simulink library "SMC"  (R2019a)
settings: Solver=VariableStepAuto  StartTime=0.0  StopTime=10.0  RelTol=1e-3
values from neighbouring files (symbols this model uses):
  A = BWB.lat.A    [Example_init.m]    (also in SMC1.m = BWB.A; SMCCanForm.m = Tr*A*Tr')
  B = BWB.lat.B    [Example_init.m]    (also in SMC1.m = BWB.B; SMCCanForm.m = Tr*B)
  CA = pinv(B2)    [SMCCanForm.m]
  Cc = [1 0 0 0 ... (first row only)    [Example_init.m]    (also in outfor.m = C*inv(Tc))
  F = -eye(2)    [Example_init.m]    (also in sqobs.m = (P2*C2*B2)')
  Lam = S*Bf    [comrobs.m]    (also in contl.m = S*B; contlCA.m = S*B; contliaCA.m = S*BT; contliaCA2.m = S*BT)
  P = lyap(Phi',eye(mm))    [comrobs.m]    (also in contl.m; contlCA.m; contliaCA.m; contliaCA2.m)
  Q = eye(4)    [Example_init.m]
  Qi = eye(2)    [Example_init.m]
settings Model: Creator=lev201  LastModifiedBy=Witali
settings DataIOCC: ReturnWorkspaceOutputs=off
settings DebuggingCC: ArithmeticOperatorsInVariantConditions=warning
settings SFSimCC: SimUseLocalCustomCode=off
settings RTWCC: RTWUseLocalCustomCode=off

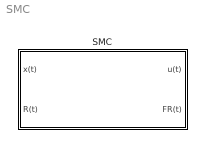
== system SMC ==
  SMC : Subsystem  mask{I=on, shs=off, adpt=off, showadpt=off, A=A, B=B, Cc=Cc, Q=Q, rho=1, C0=1, PC=1, K0=1, PK=1, delta=0.01, eps=0, Qi=Qi, Fil=on, Filter=F, FRt=on}
      mask prompts: I "Integral Action"; shs "Show s(t)"; adpt "Adaptive"; showadpt "Show Adaptive Parameters"; A "System Matrix:"; B "Effectiveness Matrix:"; Cc "Output Matrix:"; Q "State Weighting Matrix:"; C0 "Initial guess of C:"; PC "Learning rate of C estimator:"; K0 "Initial guess of K:"; PK "Learning rate of K estimator:"; delta "Sigmoidal Approximation:"; eps "Boundary Layer Thickness:"; Qi "Integral Action Weighting Matrix:"; Fil "Pre-Filter Reference Signal"; FRt "Show Filtered R(t)"
      mask init:
      | Shs=get_param(gcb, 'shs');
      | int=get_param(gcb, 'I');
      | Fil=get_param(gcb, 'fil');
      | FRT=get_param(gcb, 'FRt');
      | SAD=get_param(gcb, 'showadpt');
      | AD=get_param(gcb, 'adpt');
      | 
      | [nn mm]=size(B);
      | 
      | if strcmp(AD, 'on')
      |     rho=0; 
      |     ADPT=1;
      | else 
      |     ADPT=0;
      | end
      | 
      | if strcmp(AD, 'on') && strcmp(SAD, 'on')
      |      if strcmp(get_param([gcb '/ap(t)'], 'BlockType'), 'Terminator')
      |         replace([gcb '/ap(t)'], 'built-in/Outport');
      | %         set_param([gcb '/ap(t)'],'Port',num2str(2));
      |      end
      | else
      |     replace([gcb '/ap(t)'], 'built-in/Terminator')
      | end
      | 
      | switch int
      |     
      |     case 'off'
      |     [L, P, Lam, S, E, CA]=SMCDesign_init(A, B, Q);
      |     INTs=0;
      |     ll=size(S,1);
      |     C=zeros(ll, nn);
      |     L=[zeros(ll, ll) L];
      |     S=[zeros(ll, ll) S];
      |     Lr=[zeros(ll, ll)];
      |     
      |     case 'on'
      | 
      | 
      |         nn=size(Q,1);
      |         ll=size(Qi,1);
      |          QQ=[Qi zeros(ll, nn)
      |              zeros(nn, ll) Q];
      |        [L, Lr, P, Lam, S, E, CA]=SMCDesign_initIA(A, B, Cc, QQ);
      |        INTs=1;
      | end
      | 
      | E
      | 
      |  switch Shs
      | 
      |     case 'on'
      |         
      |         if strcmp(get_param([gcb '/s(t)'], 'BlockType'), 'Terminator')
      |         replace([gcb '/s(t)'], 'built-in/Outport');
      |         set_param([gcb '/s(t)'],'Port',num2str(2));
      |         end
      |         
      |     case 'off'
      |         
      |         if strcmp(get_param([gcb '/s(t)'], 'BlockType'),'Outport')
      |         replace([gcb '/s(t)'], 'built-in/Terminator');
      |         end
      |     
      | end
      | 
      | switch int
      |     
      |     case 'on'
      |         
      |         switch Fil
      |             
      |             case 'on'
      |                 
      |                 
      |                 replace([gcb '/r(t)'], 'built-in/Ground');
      |                 
      |                 if strcmp(get_param([gcb '/R(t)'], 'BlockType'), 'Ground')
      |                 replace([gcb '/R(t)'], 'built-in/Inport');
      |                 set_param([gcb '/R(t)'],'Port',num2str(2));
      |                 end
      |                 
      |             case 'off'
      |                 
      |                 replace([gcb '/R(t)'], 'built-in/Ground');
      |              
      |                 
      |                
      |                 if strcmp(get_param([gcb '/r(t)'], 'BlockType'), 'Ground')
      |                 replace([gcb '/r(t)'], 'built-in/Inport');
      |                 set_param([gcb '/r(t)'],'Port',num2str(2));
      |                 end
      |         end
      |         
      |     case 'off'
      |         
      |         replace([gcb '/r(t)'], 'built-in/Ground');
      |         replace([gcb '/R(t)'], 'built-in/Ground');
      | end
      | 
      | if strcmp(Fil, 'on') && strcmp(FRT, 'on') && strcmp(int, 'on')
      |      if strcmp(get_param([gcb '/FR(t)'], 'BlockType'), 'Terminator')
      |         replace([gcb '/FR(t)'], 'built-in/Outport');
      |          set_param([gcb '/FR(t)'],'Port',num2str(2));
      |      end
      | else
      |     replace([gcb '/FR(t)'], 'built-in/Terminator')
      | end
      | 
      | if strcmp(Fil, 'on') && strcmp(int, 'on')
      | 
      | else
      | 
      | Filter=zeros(ll,ll);
      | 
      | end
      mask Callback I:
      | int = get_param(gcb,'I');
      | Enables=get_param(gcb, 'MaskEnables');
      | Vis=get_param(gcb, 'MaskVisibilities');
      | 
      | 
      | if strcmp(int,'on')
      | 
      |    Enables{7}='on';
      |    Enables{16}='on';
      |    Enables{17}='on';
      |    Enables{18}='on';
      |    Enables{19}='on';
      | 
      | else
      | 
      |     Enables{7}='off';
      |    Enables{16}='off';
      |    Enables{17}='off';
      |    Enables{18}='off';
      |    Enables{19}='off';
      | 
      | 
      | end
      | set_param(gcb, 'MaskEnables', Enables)
      | set_param(gcb, 'MaskVisibilities', Vis)
      mask Callback adpt:
      | int = get_param(gcb,'adpt');
      | Enables=get_param(gcb, 'MaskEnables');
      | Vis=get_param(gcb, 'MaskVisibilities');
      | 
      | if strcmp(int,'on')
      | 
      |    Vis{4}='on';
      |    Enables{10}='on';
      |    Enables{11}='on';
      |    Enables{12}='on';
      |    Enables{13}='on';
      |    Enables{9}='off';
      | 
      | else
      | 
      |   Vis{4}='off';
      |    Enables{10}='off';
      |    Enables{11}='off';
      |    Enables{12}='off';
      |    Enables{13}='off';
      |    Enables{9}='on';
      | 
      | 
      | end
      | set_param(gcb, 'MaskEnables', Enables)
      | set_param(gcb, 'MaskVisibilities', Vis)
      mask Callback Fil:
      | FIL = get_param(gcb,'Fil');
      | Enables=get_param(gcb, 'MaskEnables');
      | Vis=get_param(gcb, 'MaskVisibilities');
      | 
      | if strcmp(FIL,'on')
      | 
      |    Vis{18}='on';
      |    Vis{19}='on';
      | 
      | else
      | 
      |    Vis{18}='off';
      |    Vis{19}='off';
      | 
      | 
      | 
      | 
      | end
      | 
      | set_param(gcb, 'MaskEnables', Enables)
      | set_param(gcb, 'MaskVisibilities', Vis)
      mask DialogControl DescGroupVar Prompt: Sliding Mode Controller
      mask DialogControl DescTextVar Prompt: Quadratic Minimisation based Sliding Mode Controller with Integral Action.
      mask DialogControl Control2 Prompt: If system is over-actuated Control Allocation is automatically used.
      mask DialogControl Container4 Prompt: Controller Configuration
      mask DialogControl Container3 Prompt: Model Parameters
      mask DialogControl Container7 Prompt: Controller Tuning
      mask DialogControl Container16 Prompt: Fixed Paramters
      mask DialogControl Container12 Prompt: Adaptive Parameters
      mask DialogControl Container8 Prompt: Chattering Avoidance
      mask DialogControl Container9 Prompt: Integral Action

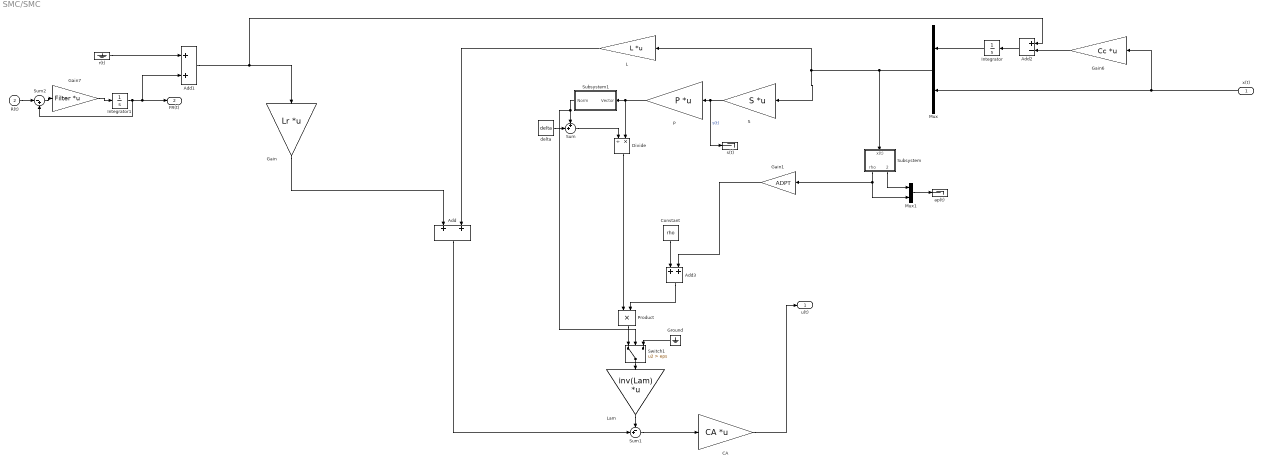
== system SMC/SMC ==
  x(t) : Inport
  R(t) : Inport  Port=2
  Add : Sum
  Add1 : Sum
  Add2 : Sum  Inputs=+-
  Add3 : Sum
  CA : Gain  Gain=CA  Multiplication=Matrix(K*u) (u vector)
  Constant : Constant  Value=rho
  Divide : Product  Inputs=/*
  Gain : Gain  Gain=Lr  Multiplication=Matrix(K*u) (u vector)
  Gain1 : Gain  Gain=ADPT
  Gain6 : Gain  Gain=Cc  Multiplication=Matrix(K*u) (u vector)
  Gain7 : Gain  Gain=Filter  Multiplication=Matrix(K*u) (u vector)
  Ground : Ground
  Integrator : Integrator
  Integrator1 : Integrator
  L : Gain  Gain=L  Multiplication=Matrix(K*u) (u vector)
  Lam : Gain  Gain=inv(Lam)  Multiplication=Matrix(K*u) (u vector)
  Mux : Mux  Inputs=2
  Mux1 : Mux  Inputs=2
  P : Gain  Gain=P  Multiplication=Matrix(K*u) (u vector)
  Product : Product
  S : Gain  Gain=S  Multiplication=Matrix(K*u) (u vector)
  Subsystem : Subsystem
  Subsystem1 : Subsystem
  Sum : Sum  Inputs=++|
  Sum1 : Sum  Inputs=-+|
  Sum2 : Sum  Inputs=|-+
  Switch1 : Switch  Criteria=u2 > Threshold  Threshold=eps  ZeroCross=off
  ap(t) : Terminator
  delta : Constant  Value=delta
  r(t) : Ground
  s(t) : Terminator
  u(t) : Outport
  FR(t) : Outport  Port=2
  wires:
  Add/1 -> Sum1/2
  Subsystem1/1(Norm) -> Switch1/2, Sum/1
  P/1 -> Divide/2, Subsystem1/1(Vector)
  Divide/1 -> Product/1
  CA/1 -> u(t)/1
  Sum1/1 -> CA/1
  Lam/1 -> Sum1/1
  S/1 -> P/1, s(t)/1  "s(t)"
  Add2/1 -> Integrator/1
  Integrator/1 -> Mux/1
  Gain6/1 -> Add2/2
  L/1 -> Add/2
  x(t)/1 -> Gain6/1, Mux/2
  Sum/1 -> Divide/1
  delta/1 -> Sum/2
  Gain/1 -> Add/1
  Mux/1 -> S/1, L/1, Subsystem/1(x(t))
  r(t)/1 -> Add1/1
  Add1/1 -> Add2/1, Gain/1
  R(t)/1 -> Sum2/1
  Sum2/1 -> Gain7/1
  Integrator1/1 -> Sum2/2, FR(t)/1, Add1/2
  Gain7/1 -> Integrator1/1
  Ground/1 -> Switch1/3
  Switch1/1 -> Lam/1
  Subsystem/2(est-par) -> Mux1/1
  Mux1/1 -> ap(t)/1
  Subsystem/1(rho) -> Gain1/1, Mux1/2
  Product/1 -> Switch1/1
  Add3/1 -> Product/2
  Constant/1 -> Add3/1
  Gain1/1 -> Add3/2

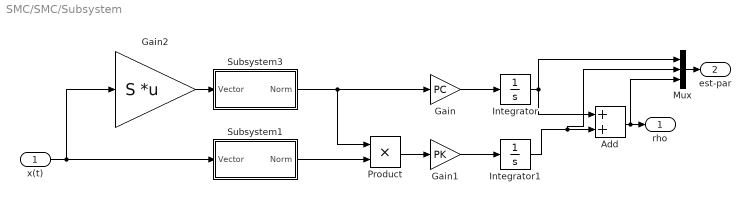
== system SMC/SMC/Subsystem ==
  x(t) : Inport
  Add : Sum
  Gain : Gain  Gain=PC
  Gain1 : Gain  Gain=PK
  Gain2 : Gain  Gain=S  Multiplication=Matrix(K*u) (u vector)
  Integrator : Integrator  InitialCondition=C0
  Integrator1 : Integrator  InitialCondition=K0
  Mux : Mux  Inputs=3
  Product : Product
  Subsystem1 : Subsystem
  Subsystem3 : Subsystem
  rho : Outport
  est-par : Outport  Port=2
  wires:
  Gain/1 -> Integrator/1
  Integrator/1 -> Add/1, Mux/1
  Subsystem3/1(Norm) -> Product/1, Gain/1
  x(t)/1 -> Subsystem1/1(Vector), Gain2/1
  Subsystem1/1(Norm) -> Product/2
  Product/1 -> Gain1/1
  Gain1/1 -> Integrator1/1
  Add/1 -> Mux/3, rho/1
  Integrator1/1 -> Mux/2, Add/2
  Gain2/1 -> Subsystem3/1(Vector)
  Mux/1 -> est-par/1

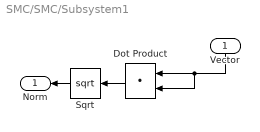
== system SMC/SMC/Subsystem1 ==
  Vector : Inport
  Dot Product : DotProduct  InputSameDT=on  OutDataTypeStr=Inherit: Inherit via internal rule
  Sqrt : Sqrt  SaturateOnIntegerOverflow=on
  Norm : Outport
  wires:
  Dot Product/1 -> Sqrt/1
  Sqrt/1 -> Norm/1
  Vector/1 -> Dot Product/2, Dot Product/1

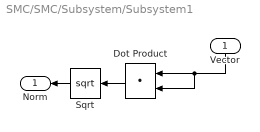
== system SMC/SMC/Subsystem/Subsystem1 ==
  Vector : Inport
  Dot Product : DotProduct  InputSameDT=on  OutDataTypeStr=Inherit: Inherit via internal rule
  Sqrt : Sqrt  SaturateOnIntegerOverflow=on
  Norm : Outport
  wires:
  Dot Product/1 -> Sqrt/1
  Sqrt/1 -> Norm/1
  Vector/1 -> Dot Product/2, Dot Product/1

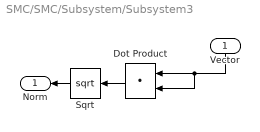
== system SMC/SMC/Subsystem/Subsystem3 ==
  Vector : Inport
  Dot Product : DotProduct  InputSameDT=on  OutDataTypeStr=Inherit: Inherit via internal rule
  Sqrt : Sqrt  SaturateOnIntegerOverflow=on
  Norm : Outport
  wires:
  Dot Product/1 -> Sqrt/1
  Sqrt/1 -> Norm/1
  Vector/1 -> Dot Product/2, Dot Product/1
